simulink model "Amatorio1"  (R2023b)
settings: Solver=VariableStepAuto  StartTime=0.0  StopTime=20  RelTol=1e-3
values from neighbouring files (symbols this model uses):
  G_den1 = [M,B,K]    [CSE_StepResponse_ME_4205_Group11_1and2_2024.m]
  G_num1 = [1]    [CSE_StepResponse_ME_4205_Group11_1and2_2024.m]
settings Model: Creator=Acer  LastModifiedBy=Acer

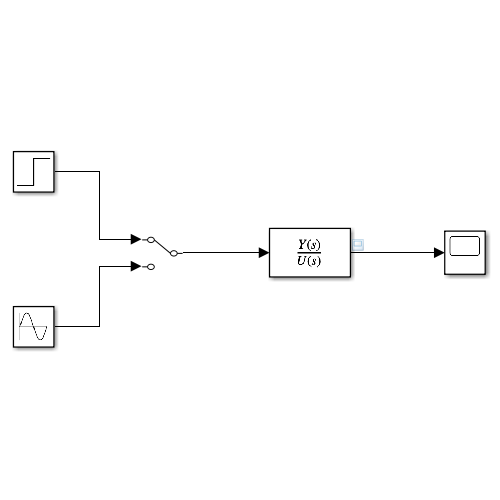
[thumbnail: Simulink's stored preview of the top-level diagram]
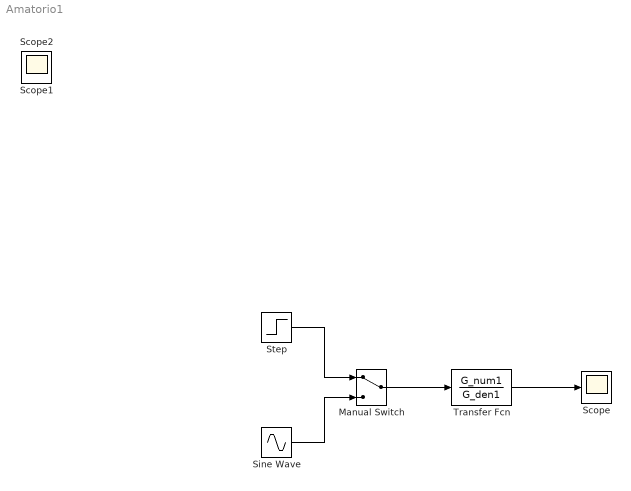
== system Amatorio1 ==
  Manual Switch : ManualSwitch
  Scope : Scope
  Sine Wave : Sin  SampleTime=0
  Step : Step  Time=0  SampleTime=0
  Transfer Fcn : TransferFcn  Numerator=G_num1  Denominator=G_den1
  Scope1 : Scope
  Scope2 : Scope
  wires:
  Sine Wave/1 -> Manual Switch/2
  Transfer Fcn/1 -> Scope/1
  Step/1 -> Manual Switch/1
  Manual Switch/1 -> Transfer Fcn/1
